simulink model "lab4_1"  (R2020a)
settings: Solver=VariableStepAuto  StartTime=0.0  StopTime=20  RelTol=1e-10  AbsTol=1e-10
values from neighbouring files (symbols this model uses):
  d_bar = (Ra/Kt)*tau_l    (= 3)    [lab4.m]
  thetades = pi / 2    (= 1.57079632679)    [lab4.m]
  Vlim = 5    [lab4.m]
libraries: cstblocks x2
settings Model: Creator=shineofanuglyjewel  LastModifiedBy=spencersun
settings DebuggingCC: SFMachineParentedDataDiag=error

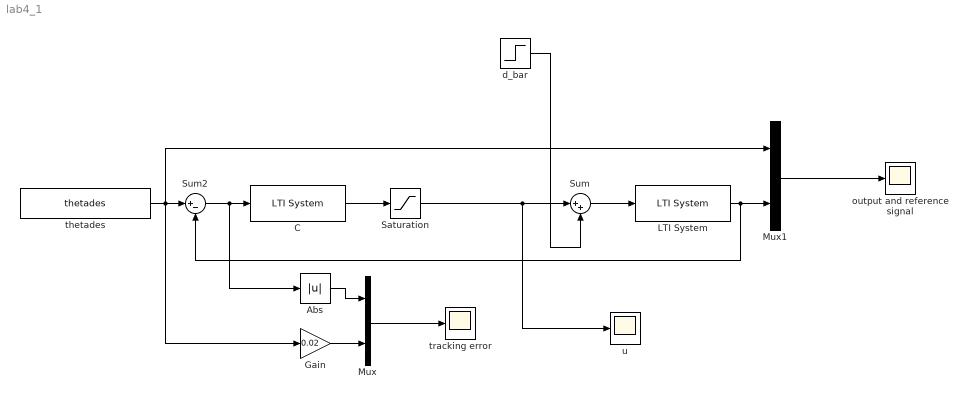
== system lab4_1 ==
  Abs : Abs
  C : cstblocks/LTI System  sys=C  IC=[]
  Gain : Gain  Gain=0.02
  LTI System : cstblocks/LTI System  sys=G  IC=[]
  Mux : Mux  Inputs=2
  Mux1 : Mux  Inputs=2
  Saturation : Saturate  UpperLimit=Vlim  LowerLimit=-Vlim
  Sum : Sum  Inputs=|++
  Sum2 : Sum  Inputs=|+-
  d_bar : Step  Time=5  After=d_bar  SampleTime=0
  output and reference signal : Scope
  thetades : Constant  Value=thetades
  tracking error : Scope
  u : Scope
  wires:
  Mux/1 -> tracking error/1
  Gain/1 -> Mux/2
  Mux1/1 -> output and reference signal/1
  Abs/1 -> Mux/1
  d_bar/1 -> Sum/2
  C/1 -> Saturation/1
  Sum/1 -> LTI System/1
  Saturation/1 -> u/1, Sum/1
  LTI System/1 -> Sum2/2, Mux1/2
  Sum2/1 -> Abs/1, C/1
  thetades/1 -> Mux1/1, Gain/1, Sum2/1
